simulink model "knee_jerk_v1"  (R2022a)
settings: Solver=VariableStepAuto  StartTime=0.0  StopTime=60  RelTol=1e-3
undefined symbols (not defined in the file): beta, K, L, M, m
settings Model: Creator=kabil  LastModifiedBy=kabil

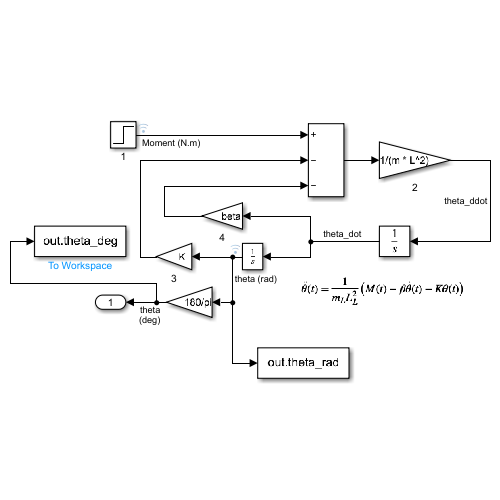
[thumbnail: Simulink's stored preview of the top-level diagram]
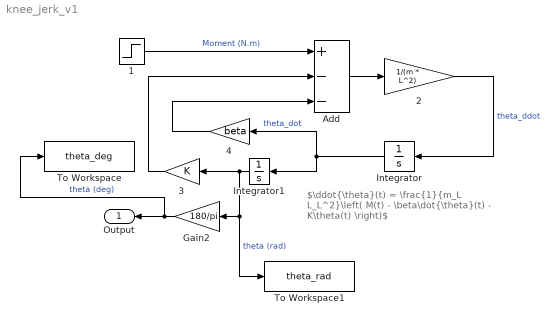
== system knee_jerk_v1 ==
  note: $\ddot{\theta}(t) = \frac{1}{m_L L_L^2}\left( M(t) - \beta\dot{\theta}(t) - K\theta(t) \right)$
  1 : Step  After=M  SampleTime=0
  2 : Gain  Gain=1/(m * L^2)
  3 : Gain  Gain=K
  4 : Gain  Gain=beta
  Add : Sum  Inputs=+--
  Gain2 : Gain  Gain=180/pi
  Integrator : Integrator
  Integrator1 : Integrator
  To Workspace : ToWorkspace  VariableName=theta_deg  SampleTime=-1
  To Workspace1 : ToWorkspace  VariableName=theta_rad  SampleTime=-1
  Output : Outport
  wires:
  Integrator/1 -> Integrator1/1, 4/1  "theta_dot"
  3/1 -> Add/2
  1/1 -> Add/1  "Moment (N.m)"
  Integrator1/1 -> 3/1, To Workspace1/1, Gain2/1  "theta (rad)"
  Add/1 -> 2/1
  4/1 -> Add/3
  2/1 -> Integrator/1  "theta_ddot"
  Gain2/1 -> To Workspace/1, Output/1  "theta (deg)"
